simulink model "ass6_workspace"  (R2020a)
settings: Solver=VariableStepAuto  StartTime=0.0  StopTime=10.0  RelTol=1e-3
values from neighbouring files (symbols this model uses):
  f_d = 0.1    [ass6.m]    (also in ass6_impedance.m)
  k_e = 1    [ass6.m]    (also in ass6_impedance.m)
  m = 1    [ass6.m]    (also in ass6_impedance.m)
  x_0 = -0.05    [ass6.m]    (also in ass6_impedance.m)
  x_d = 0.15    [ass6.m]    (also in ass6_impedance.m)
  x_dot_0 = 0    [ass6.m]    (also in ass6_impedance.m)
settings Model: Creator=sheld  LastModifiedBy=sheld

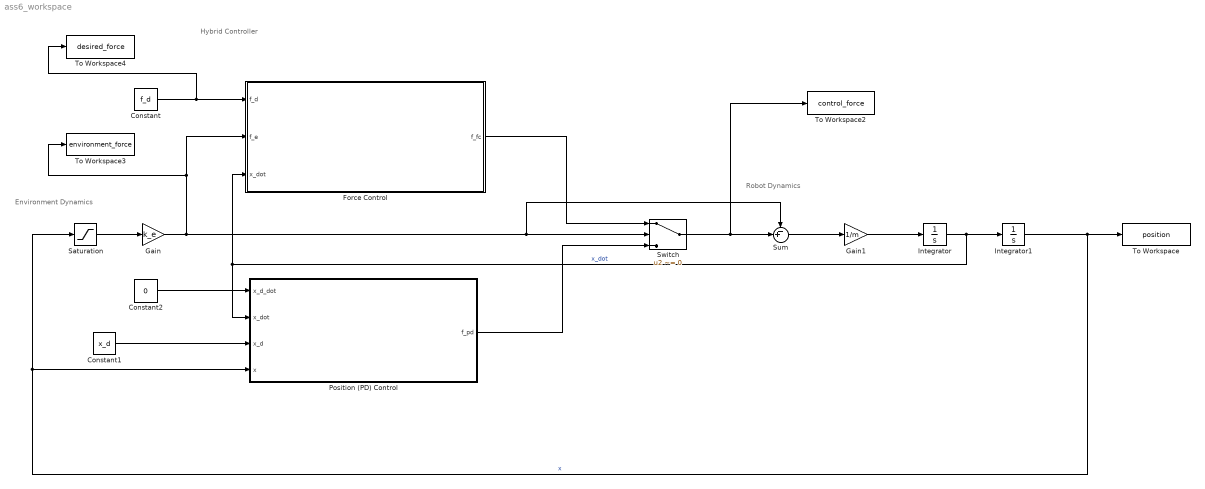
== system ass6_workspace ==
  note: Robot Dynamics
  note: Environment Dynamics
  note: Hybrid Controller
  Constant : Constant  Value=f_d
  Constant1 : Constant  Value=x_d
  Constant2 : Constant  Value=0
  Force Control : MATLAB Function  TreatAsAtomicUnit=on
  Gain : Gain  Gain=k_e
  Gain1 : Gain  Gain=1/m
  Integrator : Integrator  InitialCondition=x_dot_0
  Integrator1 : Integrator  InitialCondition=x_0
  Position (PD) Control : MATLAB Function  TreatAsAtomicUnit=on
  Saturation : Saturate  UpperLimit=inf  LowerLimit=0
  Sum : Sum  Inputs=-+|
  Switch : Switch  Criteria=u2 ~= 0
  To Workspace : ToWorkspace  VariableName=position  SampleTime=-1
  To Workspace2 : ToWorkspace  VariableName=control_force  SampleTime=-1
  To Workspace3 : ToWorkspace  VariableName=environment_force  SampleTime=-1
  To Workspace4 : ToWorkspace  VariableName=desired_force  SampleTime=-1
  wires:
  Force Control/1(f_fc) -> Switch/1
  Position (PD) Control/1(f_pd) -> Switch/3
  Gain/1 -> Switch/2, Sum/1, To Workspace3/1, Force Control/2(f_e)
  Saturation/1 -> Gain/1
  Constant2/1 -> Position (PD) Control/1(x_d_dot)
  Constant/1 -> To Workspace4/1, Force Control/1(f_d)
  Constant1/1 -> Position (PD) Control/3(x_d)
  Switch/1 -> To Workspace2/1, Sum/2
  Sum/1 -> Gain1/1
  Gain1/1 -> Integrator/1
  Integrator/1 -> Force Control/3(x_dot), Position (PD) Control/2(x_dot), Integrator1/1  "x_dot"
  Integrator1/1 -> To Workspace/1, Position (PD) Control/4(x), Saturation/1  "x"

== matlab function ass6_workspace/Position (PD) Control ==
  data: x_d_dot input; x_dot input; f_pd output; x_d input; x input
function f_pd = fcn(x_d_dot, x_dot, x_d, x)

% Assumption: step response => x_d_dot = 0
x_d_dot = 0;

% Controller gains
k_px = 5.29;
k_dx = 4.6;

f_pd = k_dx*(x_d_dot - x_dot) + k_px*(x_d - x);

== matlab function ass6_workspace/Force Control ==
  data: f_d input; f_fc output; f_e input; x_dot input
function f_fc = fcn(f_d, f_e, x_dot)

% Constants
m = 1;
k_e = 1;

% Controller gains
k_pf = 4.29;
k_vf = 4.6;

e_f = f_d - f_e;
f_fc = m*(1/k_e*k_pf*e_f - k_vf*x_dot) + f_d;
